simulink model "sp_sim"  (R2021b)
settings: Solver=VariableStepAuto  StartTime=0.0  StopTime=60  MaxStep=0.01  RelTol=1e-3  EnableMultiTasking=on
StopFcn:
  | figure(1)
  | 
  | subplot(411);
  | plot(y1.time,y1.data,y2.time,y2.data,'LineWidth',2)
  | hold on; plot(r.time,r.data,'k--'); hold off
  | %ylim([-2 3]);
  | title('Réponses avec PID et Prédicteur de Smith');
  | ylabel('r(t) , y(t)');
  | xlabel('Temps (s)');
  | legend('y1','y2','r');
  | grid on
  | 
  | subplot(412);
  | plot(u1.time,u1.data,u2.time,u2.data,'LineWidth',2)
  | ylim([-0.5 1]);
  | ylabel('u(t)');
  | xlabel('Temps (s)');
  | legend('u1','u2','r');
  | grid on
  | 
  | subplot(413);
  | plot(e1.time,e1.data,e2.time,e2.data,em.time,em.data,'LineWidth',2)
  | ylim([-1 2]);
  | ylabel('u(t)');
  | xlabel('Temps (s)');
  | legend('e1','e2','em');
  | grid on
  | 
  | subplot(414);
  | plot(yms.time,yms.data,'LineWidth',2)
  | hold on; plot(rs.time,rs.data,'k--'); hold off
  | ylim([-1 2]);
  | ylabel('u(t)');
  | xlabel('Temps (s)');
  | legend('yms','rs');
  | grid on
  | 
  | set(gcf,'Position',[100 100 500 700])
  | saveas(gcf,'ex4_11_respplots.png')
values from neighbouring files (symbols this model uses):
  Km = Kp    (= 5)    [sp_vs_pid.m]
  T1m = T1    (= 5)    [sp_vs_pid.m]
  theta = 10    [sp_vs_pid.m]
  theta_m = theta    (= 10)    [sp_vs_pid.m]
undefined symbols (not defined in the file or in its folder): KcPID, KcSP, Td, Tf, Ti
libraries: cstblocks x2
settings Model: Creator=LiberT  LastModifiedBy=billtubbs
settings SolverCC: AlgebraicLoopSolver=TrustRegion
settings DataIOCC: LimitDataPoints=on  SaveFormat=Array  SignalLoggingSaveFormat=ModelDataLogs  SaveTime=off  ReturnWorkspaceOutputs=off
settings OptimizationCC: BooleanDataType=off  ExpressionDepthLimit=2147483647  InitFltsAndDblsToZero=on  LifeSpan=inf
settings DebuggingCC: SaveWithParameterizedLinksMsg=none  UnderspecifiedInitializationDetection=Classic  MergeDetectMultiDrivingBlocksExec=none  SignalResolutionControl=TryResolveAllWithWarning  MultiTaskDSMMsg=warning  MultiTaskCondExecSysMsg=none  FcnCallInpInsideContextMsg=warning  StateNameClashWarn=warning  SFUnexpectedBacktrackingDiag=warning  SFNoUnconditionalDefaultTransitionDiag=warning  SFExecutionAtInitializationDiag=none  SFMachineParentedDataDiag=warning  ArithmeticOperatorsInVariantConditions=warning
settings HardwareCC: ProdBitPerPointer=32  ProdBitPerSizeT=32  ProdBitPerPtrDiffT=32  ProdLargestAtomicFloat=None  ProdIntDivRoundTo=Undefined  ProdEndianess=Unspecified  ProdWordSize=32  ProdHWDeviceType=32-bit Generic  TargetBitPerLong=64  TargetBitPerPointer=64  TargetBitPerSizeT=64  TargetBitPerPtrDiffT=64  TargetLongLongMode=on  TargetIntDivRoundTo=Zero  TargetEndianess=LittleEndian  TargetWordSize=64  TargetHWDeviceType=MATLAB Host  ProdEqTarget=off
settings ModelReferenceCC: PropagateSignalLabelsOutOfModel=off
settings SFSimCC: SimUseLocalCustomCode=off  CustomCodeUndefinedFunction=UseInterfaceOnly
settings RTWCC: RTWUseLocalCustomCode=off
settings CodeAppCC: StateflowObjectComments=on
settings GRTTargetCC: TargetFcnLib=ansi_tfl_tmw.mat  TargetLangStandard=C89/C90 (ANSI)  ModelReferenceCompliant=off  CombineOutputUpdateFcns=off  MatFileLogging=off  GRTInterface=on
settings ConfigComp: CovMetricSettings=dw  CovSaveCumulativeToWorkspaceVar=on  CovSaveSingleToWorkspaceVar=on  CovExternalEMLEnable=off  CovSFcnEnable=off

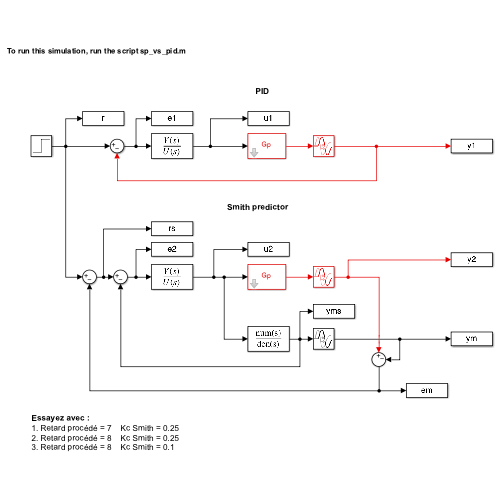
[thumbnail: Simulink's stored preview of the top-level diagram]
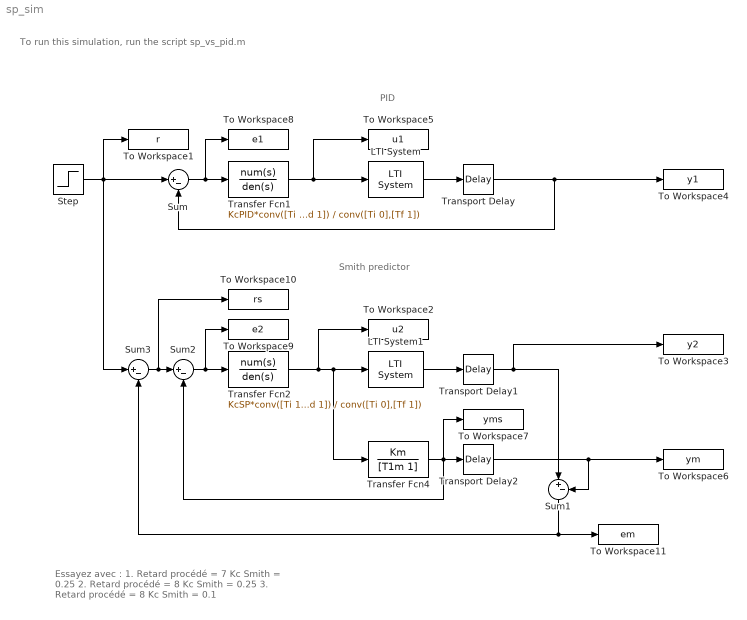
== system sp_sim ==
  note: To run this simulation, run the script sp_vs_pid.m
  note: Essayez avec :
      | 1. Retard procédé = 7 Kc Smith = 0.25
      | 2. Retard procédé = 8 Kc Smith = 0.25
      | 3. Retard procédé = 8 Kc Smith = 0.1
  note: PID
  note: Smith predictor
  LTI System : cstblocks/LTI System  sys=Gp  IC=[]
  LTI System1 : cstblocks/LTI System  sys=Gp  IC=[]
  Step : Step  SampleTime=0
  Sum{,1..3} (4 alike) : Sum  Inputs=|+-  InputSameDT=on  SaturateOnIntegerOverflow=on  OutDataTypeStr=Inherit: Same as first input
  To Workspace1 : ToWorkspace  VariableName=r  SaveFormat=Timeseries  SampleTime=-1
  To Workspace10 : ToWorkspace  VariableName=rs  SaveFormat=Timeseries  SampleTime=-1
  To Workspace11 : ToWorkspace  VariableName=em  SaveFormat=Timeseries  SampleTime=-1
  To Workspace2 : ToWorkspace  VariableName=u2  SaveFormat=Timeseries  SampleTime=-1
  To Workspace3 : ToWorkspace  VariableName=y2  SaveFormat=Timeseries  SampleTime=-1
  To Workspace4 : ToWorkspace  VariableName=y1  SaveFormat=Timeseries  SampleTime=-1
  To Workspace5 : ToWorkspace  VariableName=u1  SaveFormat=Timeseries  SampleTime=-1
  To Workspace6 : ToWorkspace  VariableName=ym  SaveFormat=Timeseries  SampleTime=-1
  To Workspace7 : ToWorkspace  VariableName=yms  SaveFormat=Timeseries  SampleTime=-1
  To Workspace8 : ToWorkspace  VariableName=e1  SaveFormat=Timeseries  SampleTime=-1
  To Workspace9 : ToWorkspace  VariableName=e2  SaveFormat=Timeseries  SampleTime=-1
  Transfer Fcn1 : TransferFcn  Numerator=KcPID*conv([Ti 1],[Td 1])  Denominator=conv([Ti 0],[Tf 1])
  Transfer Fcn2 : TransferFcn  Numerator=KcSP*conv([Ti 1],[Td 1])  Denominator=conv([Ti 0],[Tf 1])
  Transfer Fcn4 : TransferFcn  Numerator=Km  Denominator=[T1m 1]
  Transport Delay : TransportDelay  DelayTime=theta
  Transport Delay1 : TransportDelay  DelayTime=theta
  Transport Delay2 : TransportDelay  DelayTime=theta_m
  wires:
  Step/1 -> Sum3/1, To Workspace1/1, Sum/1
  Sum/1 -> To Workspace8/1, Transfer Fcn1/1
  Transfer Fcn1/1 -> LTI System/1, To Workspace5/1
  LTI System/1 -> Transport Delay/1
  Transport Delay/1 -> Sum/2, To Workspace4/1
  LTI System1/1 -> Transport Delay1/1
  Transfer Fcn4/1 -> Sum2/2, To Workspace7/1, Transport Delay2/1
  Transfer Fcn2/1 -> LTI System1/1, Transfer Fcn4/1, To Workspace2/1
  Transport Delay1/1 -> Sum1/1, To Workspace3/1
  Transport Delay2/1 -> To Workspace6/1, Sum1/2
  Sum2/1 -> To Workspace9/1, Transfer Fcn2/1
  Sum3/1 -> To Workspace10/1, Sum2/1
  Sum1/1 -> Sum3/2, To Workspace11/1
